simulink model "MBD_Arnav2020b"  (R2020b)
settings: Solver=FixedStepAuto  StartTime=0.0  StopTime=inf  FixedStep=1  RelTol=1e-3
undefined symbols (not defined in the file): sigbuilder_block
settings Model: Creator=99003730  LastModifiedBy=99003730

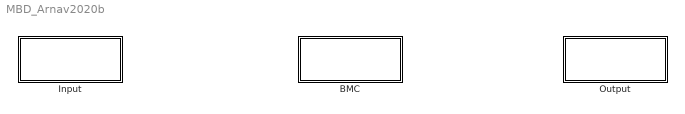
== system MBD_Arnav2020b ==
  BMC : Subsystem
  Input : Subsystem
  Output : Subsystem

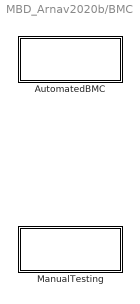
== system MBD_Arnav2020b/BMC ==
  AutomatedBMC : Subsystem
  ManualTesting : Subsystem

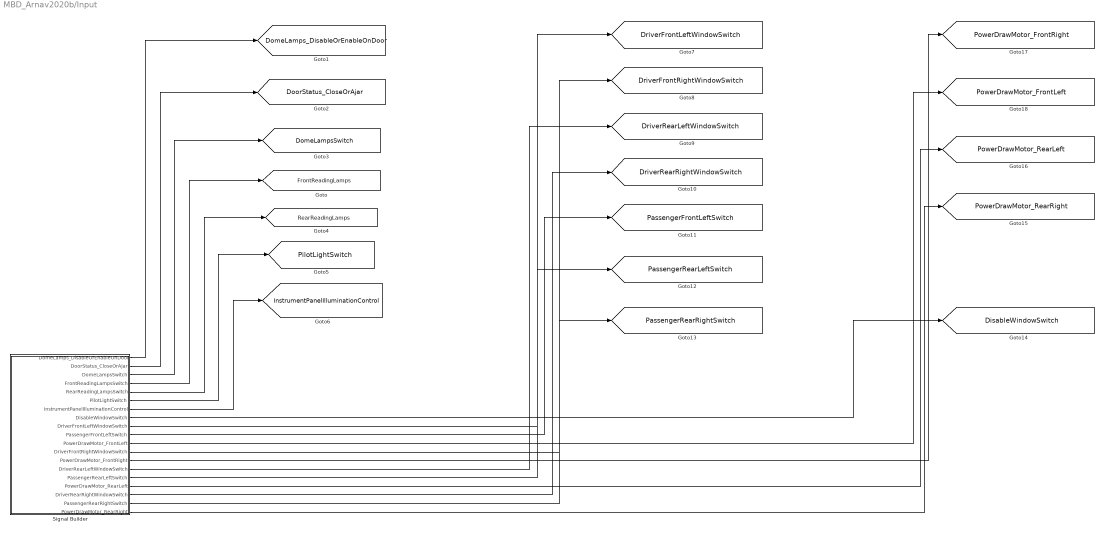
== system MBD_Arnav2020b/Input ==
  Signal Builder : Subsystem  Tag=STV Subsys  LoadFcn=sigbuilder_block('load');  StartFcn=sigbuilder_block('start');  StopFcn=sigbuilder_block('stop');  ClipboardFcn=sigbuilder_block('clipboard');  mask(Sigbuilder block){tuvar=[0:10]}
      mask help: Simulink:masks:SigbuilderBlock_MD
      mask init:
      | if ~strcmp(get_param(bdroot(gcbh),'SimulationStatus'),'stopped') tuvar = sigbuilder_block('maskInit'); end
      settings: CopyFcn=sigbuilder_block('copy');  DeleteFcn=sigbuilder_block('delete');  ModelCloseFcn=sigbuilder_block('modelClose');  PreSaveFcn=sigbuilder_block('preSave');  PauseFcn=sigbuilder_block('pause');  ContinueFcn=sigbuilder_block('continue');  NameChangeFcn=sigbuilder_block('namechange');  OpenFcn=sigbuilder_block('open',[6 80.25 1188 465.75 ]);  CloseFcn=sigbuilder_block('close');
      mask Display: plot(0, 0, 100, 100,[2, 2, 32, 32, 2], [68, 8, 8, 68, 68],[32, 2], [38, 38], [32, 19, 2],[53, 60, 44], [32, 17, 17, 2],[16, 16, 31, 31]);txt = getActiveGroup(gcbh);text(2, 100, txt,'verticalAlignment', 'top');
  tag scope: DisableWindowSwitch=global, DomeLampsSwitch=global, DomeLamps_DisableOrEnableOnDoor=global, DoorStatus_CloseOrAjar=global, DriverFrontLeftWindowSwitch=global, DriverFrontRightWindowSwitch=global, DriverRearLeftWindowSwitch=global, DriverRearRightWindowSwitch=global, FrontReadingLamps=global, InstrumentPanelIlluminationControl=global, PassengerFrontLeftSwitch=global, PassengerRearLeftSwitch=global, PassengerRearRightSwitch=global, PilotLightSwitch=global, PowerDrawMotor_FrontLeft=global, PowerDrawMotor_FrontRight=global, PowerDrawMotor_RearLeft=global, PowerDrawMotor_RearRight=global, RearReadingLamps=global
  wires:
  Signal Builder/9(DriverFrontLeftWindowSwitch) -> [DriverFrontLeftWindowSwitch]
  Signal Builder/12(DriverFrontRightWindowSwitch) -> [DriverFrontRightWindowSwitch]
  Signal Builder/14(DriverRearLeftWindowSwitch) -> [DriverRearLeftWindowSwitch]
  Signal Builder/17(DriverRearRightWindowSwitch) -> [DriverRearRightWindowSwitch]
  Signal Builder/10(PassengerFrontLeftSwitch) -> [PassengerFrontLeftSwitch]
  Signal Builder/15(PassengerRearLeftSwitch) -> [PassengerRearLeftSwitch]
  Signal Builder/18(PassengerRearRightSwitch) -> [PassengerRearRightSwitch]
  Signal Builder/13(PowerDrawMotor_FrontRight) -> [PowerDrawMotor_FrontRight]
  Signal Builder/11(PowerDrawMotor_FrontLeft) -> [PowerDrawMotor_FrontLeft]
  Signal Builder/16(PowerDrawMotor_RearLeft) -> [PowerDrawMotor_RearLeft]
  Signal Builder/19(PowerDrawMotor_RearRight) -> [PowerDrawMotor_RearRight]
  Signal Builder/8(DisableWindowSwitch) -> [DisableWindowSwitch]
  Signal Builder/1(DomeLamps_DisableOrEnableOnDoor) -> [DomeLamps_DisableOrEnableOnDoor]
  Signal Builder/2(DoorStatus_CloseOrAjar) -> [DoorStatus_CloseOrAjar]
  Signal Builder/3(DomeLampsSwitch) -> [DomeLampsSwitch]
  Signal Builder/4(FrontReadingLampsSwitch) -> [FrontReadingLamps]
  Signal Builder/5(RearReadingLampsSwitch) -> [RearReadingLamps]
  Signal Builder/6(PilotLightSwitch) -> [PilotLightSwitch]
  Signal Builder/7(InstrumentPanelIlluminationControl) -> [InstrumentPanelIlluminationControl]

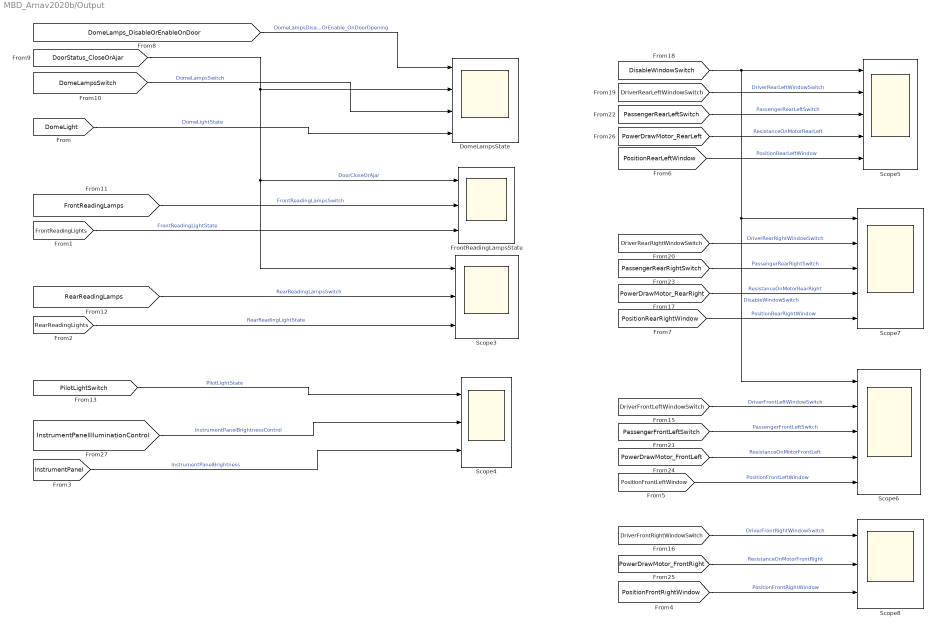
== system MBD_Arnav2020b/Output ==
  DomeLampsState : Scope  NumInputPorts=4
  FrontReadingLampsState : Scope  NumInputPorts=3
  Scope3 : Scope  NumInputPorts=3
  Scope4 : Scope  NumInputPorts=3
  Scope5 : Scope  NumInputPorts=5
  Scope6 : Scope  NumInputPorts=5
  Scope7 : Scope  NumInputPorts=5
  Scope8 : Scope  NumInputPorts=3
  wires:
  [RearReadingLights] -> Scope3/3  "RearReadingLightState"
  [FrontReadingLights] -> FrontReadingLampsState/3  "FrontReadingLightState"
  [DomeLight] -> DomeLampsState/4  "DomeLightState"
  [InstrumentPanel] -> Scope4/3  "InstrumentPanelBrightness"
  [PositionRearLeftWindow] -> Scope5/5  "PositionRearLeftWindow"
  [DomeLamps_DisableOrEnableOnDoor] -> DomeLampsState/1  "DomeLampsDisableOrEnable_OnDoorOpening"
  [DoorStatus_CloseOrAjar] -> Scope3/1, FrontReadingLampsState/1, DomeLampsState/2  "DoorCloseOrAjar"
  [DomeLampsSwitch] -> DomeLampsState/3  "DomeLampsSwitch"
  [FrontReadingLamps] -> FrontReadingLampsState/2  "FrontReadingLampsSwitch"
  [RearReadingLamps] -> Scope3/2  "RearReadingLampsSwitch"
  [PilotLightSwitch] -> Scope4/1  "PilotLightState"
  [InstrumentPanelIlluminationControl] -> Scope4/2  "InstrumentPanelBrightnessControl"
  [DisableWindowSwitch] -> Scope6/1, Scope7/1, Scope5/1  "DisableWindowSwitch"
  [DriverRearLeftWindowSwitch] -> Scope5/2  "DriverRearLeftWindowSwitch"
  [PassengerRearLeftSwitch] -> Scope5/3  "PassengerRearLeftSwitch"
  [PowerDrawMotor_RearLeft] -> Scope5/4  "ResistanceOnMotorRearLeft"
  [DriverRearRightWindowSwitch] -> Scope7/2  "DriverRearRightWindowSwitch"
  [PassengerRearRightSwitch] -> Scope7/3  "PassengerRearRightSwitch"
  [PowerDrawMotor_RearRight] -> Scope7/4  "ResistanceOnMotorRearRight"
  [PositionRearRightWindow] -> Scope7/5  "PositionRearRightWindow"
  [DriverFrontLeftWindowSwitch] -> Scope6/2  "DriverFrontLeftWindowSwitch"
  [PassengerFrontLeftSwitch] -> Scope6/3  "PassengerFrontLeftSwitch"
  [PowerDrawMotor_FrontLeft] -> Scope6/4  "ResistanceOnMotorFrontLeft"
  [PositionFrontLeftWindow] -> Scope6/5  "PositionFrontLeftWindow"
  [DriverFrontRightWindowSwitch] -> Scope8/1  "DriverFrontRightWindowSwitch"
  [PowerDrawMotor_FrontRight] -> Scope8/2  "ResistanceOnMotorFrontRight"
  [PositionFrontRightWindow] -> Scope8/3  "PositionFrontRightWindow"

== system MBD_Arnav2020b/BMC/AutomatedBMC ==
  "Arnav's Subsytem (Interior Lighting and power windows) " : Subsystem

== system MBD_Arnav2020b/BMC/ManualTesting ==
  Manual Testing Arnav : Subsystem

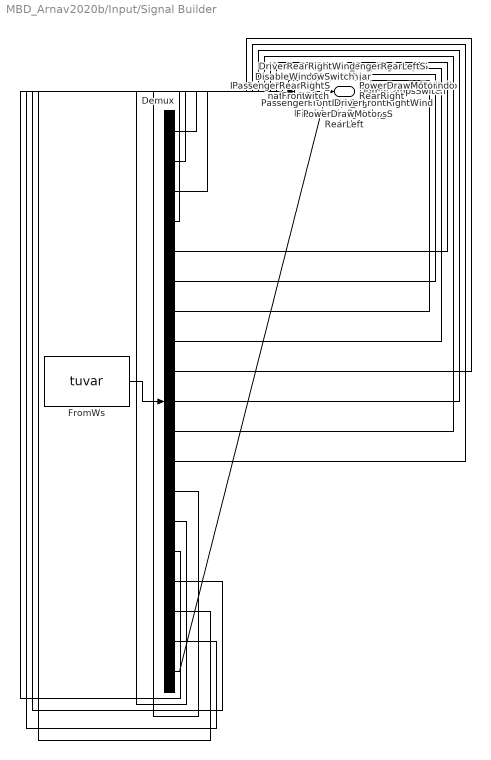
== system MBD_Arnav2020b/Input/Signal Builder ==
  Demux : Demux  Tag=STV Demux  Outputs=19
      settings: DisplayOption=none
  FromWs : FromWorkspace  Tag=STV FromWs  VariableName=tuvar  SampleTime=1
      SigBuilderData=|
      | common.afterFinalStr = 'Extrapolate'
      | common.sampleTime = '1'
      | dataSet.timeRange = [0 25]
      | dataSet.name = 'Sheet1'
      | sbobj.Name = 'Signal Builder'
      | sbobj.Groups.Name = 'Sheet1'
      | sbobj.Groups.Signals(1).Name = 'DomeLamps_DisableOrEnableOnDoor'
      | sbobj.Groups.Signals(1).XData = [0 1 2 3 4 5 6 7 8 9 10 11 12 13 14 15 16 17 18 19 20 21 22 23 24 25]
      | sbobj.Groups.Signals(1).YData = [0 0 0 0 1 1 1 1 0 0 0 0 1 1 1 1 0 0 0 0 1 1 1 1 1 0]
      | sbobj.Groups.Signals(2).Name = 'DoorStatus_CloseOrAjar'
      | sbobj.Groups.Signals(2).XData = [0 1 2 3 4 5 6 7 8 9 10 11 12 13 14 15 16 17 18 19 20 21 22 23 24 25]
      | sbobj.Groups.Signals(2).YData = [0 0 1 1 0 0 0 1 0 0 1 1 0 0 1 1 0 0 1 1 0 0 1 1 1 0]
      | sbobj.Groups.Signals(3).Name = 'DomeLampsSwitch'
      | sbobj.Groups.Signals(3).XData = [0 1 2 3 4 5 6 7 8 9 10 11 12 13 14 15 16 17 18 19 20 21 22 23 24 25]
      | sbobj.Groups.Signals(3).YData = [0 1 0 1 0 0 0 1 0 0 0 1 0 1 0 1 0 1 0 1 0 1 0 1 1 0]
      | sbobj.Groups.Signals(4).Name = 'FrontReadingLampsSwitch'
      | sbobj.Groups.Signals(4).XData = [0 1 2 3 4 5 6 7 8 9 10 11 12 13 14 15 16 17 18 19 20 21 22 23 24 25]
      | sbobj.Groups.Signals(4).YData = [0 1 0 1 0 1 0 1 0 1 0 1 0 1 0 1 0 1 0 1 0 1 0 1 0 1]
      | sbobj.Groups.Signals(5).Name = 'RearReadingLampsSwitch'
      | sbobj.Groups.Signals(5).XData = [0 1 2 3 4 5 6 7 8 9 10 11 12 13 14 15 16 17 18 19 20 21 22 23 24 25]
      | sbobj.Groups.Signals(5).YData = [0 1 0 1 0 1 0 1 0 1 0 1 0 1 0 1 0 1 0 1 0 1 0 1 0 1]
      | sbobj.Groups.Signals(6).Name = 'PilotLightSwitch'
      | sbobj.Groups.Signals(6).XData = [0 1 2 3 4 5 6 7 8 9 10 11 12 13 14 15 16 17 18 19 20 21 22 23 24 25]
      | sbobj.Groups.Signals(6).YData = [0 0 0 0 0 0 0 0 0 0 1 1 1 1 1 1 1 1 1 1 0 0 0 0 0 0]
      | sbobj.Groups.Signals(7).Name = 'InstrumentPanelIlluminationControl'
      | sbobj.Groups.Signals(7).XData = [0 1 2 3 4 5 6 7 8 9 10 11 12 13 14 15 16 17 18 19 20 21 22 23 24 25]
      | sbobj.Groups.Signals(7).YData = [1 2 3 4 5 6 7 8 9 10 1 2 3 4 5 6 7 8 9 10 1 2 3 4 5 6]
      | sbobj.Groups.Signals(8).Name = 'DisableWindowSwitch'
      | sbobj.Groups.Signals(8).XData = [0 1 2 3 4 5 6 7 8 9 10 11 12 13 14 15 16 17 18 19 20 21 22 23 24 25]
      | sbobj.Groups.Signals(8).YData = [0 0 0 0 0 0 0 0 0 0 0 0 0 0 0 0 0 1 1 0 1 1 1 0 0 0]
      | sbobj.Groups.Signals(9).Name = 'DriverFrontLeftWindowSwitch'
      | sbobj.Groups.Signals(9).XData = [0 1 2 3 4 5 6 7 8 9 10 11 12 13 14 15 16 17 18 19 20 21 22 23 24 25]
      | sbobj.Groups.Signals(9).YData = [1 1 1 0 0 0 0 0 -1 -1 -1 0 0 2 0 0 0 0 -2 0 0 0 0 0 1 0]
      | sbobj.Groups.Signals(10).Name = 'PassengerFrontLeftSwitch'
      | sbobj.Groups.Signals(10).XData = [0 1 2 3 4 5 6 7 8 9 10 11 12 13 14 15 16 17 18 19 20 21 22 23 24 25]
      | sbobj.Groups.Signals(10).YData = [0 -1 -1 1 1 1 -1 -1 0 0 0 0 0 0 0 -2 1 2 0 2 1 1 0 2 0 0]
      | sbobj.Groups.Signals(11).Name = 'PowerDrawMotor_FrontLeft'
      | sbobj.Groups.Signals(11).XData = [0 1 2 3 4 5 6 7 8 9 10 11 12 13 14 15 16 17 18 19 20 21 22 23 24 25]
      | sbobj.Groups.Signals(11).YData = [2 2 2 2 2 2 2 2 2 2 2 2 2 2 2 2 2 2 2 2 2 4 1 1 1 1]
      | sbobj.Groups.Signals(12).Name = 'DriverFrontRightWindowSwitch'
      | sbobj.Groups.Signals(12).XData = [0 1 2 3 4 5 6 7 8 9 10 11 12 13 14 15 16 17 18 19 20 21 22 23 24 25]
      | sbobj.Groups.Signals(12).YData = [1 1 1 1 1 0 0 0 -1 -1 -1 0 0 2 0 0 0 0 -2 0 0 0 0 1 2 0]
      | sbobj.Groups.Signals(13).Name = 'PowerDrawMotor_FrontRight'
      | sbobj.Groups.Signals(13).XData = [0 1 2 3 4 5 6 7 8 9 10 11 12 13 14 15 16 17 18 19 20 21 22 23 24 25]
      | sbobj.Groups.Signals(13).YData = [2 2 2 2 2 2 2 2 2 2 2 2 2 2 2 2 2 2 2 2 2 4 1 1 1 1]
      | sbobj.Groups.Signals(14).Name = 'DriverRearLeftWindowSwitch'
      | sbobj.Groups.Signals(14).XData = [0 1 2 3 4 5 6 7 8 9 10 11 12 13 14 15 16 17 18 19 20 21 22 23 24 25]
      | sbobj.Groups.Signals(14).YData = [1 1 1 0 0 0 0 0 -1 -1 -1 0 0 2 0 0 0 0 -2 0 0 0 0 0 0 0]
      | sbobj.Groups.Signals(15).Name = 'PassengerRearLeftSwitch'
      | sbobj.Groups.Signals(15).XData = [0 1 2 3 4 5 6 7 8 9 10 11 12 13 14 15 16 17 18 19 20 21 22 23 24 25]
      | sbobj.Groups.Signals(15).YData = [0 -1 -1 1 1 1 -1 -1 0 0 0 0 0 0 0 -2 1 2 0 2 1 1 0 2 0 0]
      | sbobj.Groups.Signals(16).Name = 'PowerDrawMotor_RearLeft'
      | sbobj.Groups.Signals(16).XData = [0 1 2 3 4 5 6 7 8 9 10 11 12 13 14 15 16 17 18 19 20 21 22 23 24 25]
      | sbobj.Groups.Signals(16).YData = [2 2 2 2 2 2 2 2 2 2 2 2 2 2 2 2 2 2 2 2 2 4 1 1 1 1]
      | sbobj.Groups.Signals(17).Name = 'DriverRearRightWindowSwitch'
      | sbobj.Groups.Signals(17).XData = [0 1 2 3 4 5 6 7 8 9 10 11 12 13 14 15 16 17 18 19 20 21 22 23 24 25]
      | sbobj.Groups.Signals(17).YData = [1 1 1 0 0 0 0 0 -1 -1 -1 0 0 2 0 0 0 0 -2 0 0 0 0 0 0 0]
      | sbobj.Groups.Signals(18).Name = 'PassengerRearRightSwitch'
      | sbobj.Groups.Signals(18).XData = [0 1 2 3 4 5 6 7 8 9 10 11 12 13 14 15 16 17 18 19 20 21 22 23 24 25]
      | sbobj.Groups.Signals(18).YData = [0 -1 -1 1 1 1 -1 -1 0 0 0 0 0 0 0 -2 1 2 0 2 1 1 0 2 0 0]
      | sbobj.Groups.Signals(19).Name = 'PowerDrawMotor_RearRight'
      | sbobj.Groups.Signals(19).XData = [0 1 2 3 4 5 6 7 8 9 10 11 12 13 14 15 16 17 18 19 20 21 22 23 24 25]
      | sbobj.Groups.Signals(19).YData = [2 2 2 4 2 2 2 2 2 2 2 2 2 2 2 2 2 2 4 2 2 4 1 1 1 1]
      | sbobj.Groups.TimeRange = [0 25]
  DomeLamps_DisableOrEnableOnDoor : Outport  Tag=STV Outport
  DoorStatus_CloseOrAjar : Outport  Tag=STV Outport  Port=2
  DomeLampsSwitch : Outport  Tag=STV Outport  Port=3
  FrontReadingLampsSwitch : Outport  Tag=STV Outport  Port=4
  RearReadingLampsSwitch : Outport  Tag=STV Outport  Port=5
  PilotLightSwitch : Outport  Tag=STV Outport  Port=6
  InstrumentPanelIlluminationControl : Outport  Tag=STV Outport  Port=7
  DisableWindowSwitch : Outport  Tag=STV Outport  Port=8
  DriverFrontLeftWindowSwitch : Outport  Tag=STV Outport  Port=9
  PassengerFrontLeftSwitch : Outport  Tag=STV Outport  Port=10
  PowerDrawMotor_FrontLeft : Outport  Tag=STV Outport  Port=11
  DriverFrontRightWindowSwitch : Outport  Tag=STV Outport  Port=12
  PowerDrawMotor_FrontRight : Outport  Tag=STV Outport  Port=13
  DriverRearLeftWindowSwitch : Outport  Tag=STV Outport  Port=14
  PassengerRearLeftSwitch : Outport  Tag=STV Outport  Port=15
  PowerDrawMotor_RearLeft : Outport  Tag=STV Outport  Port=16
  DriverRearRightWindowSwitch : Outport  Tag=STV Outport  Port=17
  PassengerRearRightSwitch : Outport  Tag=STV Outport  Port=18
  PowerDrawMotor_RearRight : Outport  Tag=STV Outport  Port=19
  wires:
  FromWs/1 -> Demux/1
  Demux/1 -> DomeLamps_DisableOrEnableOnDoor/1
  Demux/2 -> DoorStatus_CloseOrAjar/1
  Demux/3 -> DomeLampsSwitch/1
  Demux/4 -> FrontReadingLampsSwitch/1
  Demux/5 -> RearReadingLampsSwitch/1
  Demux/6 -> PilotLightSwitch/1
  Demux/7 -> InstrumentPanelIlluminationControl/1
  Demux/8 -> DisableWindowSwitch/1
  Demux/9 -> DriverFrontLeftWindowSwitch/1
  Demux/10 -> PassengerFrontLeftSwitch/1
  Demux/11 -> PowerDrawMotor_FrontLeft/1
  Demux/12 -> DriverFrontRightWindowSwitch/1
  Demux/13 -> PowerDrawMotor_FrontRight/1
  Demux/14 -> DriverRearLeftWindowSwitch/1
  Demux/15 -> PassengerRearLeftSwitch/1
  Demux/16 -> PowerDrawMotor_RearLeft/1
  Demux/17 -> DriverRearRightWindowSwitch/1
  Demux/18 -> PassengerRearRightSwitch/1
  Demux/19 -> PowerDrawMotor_RearRight/1

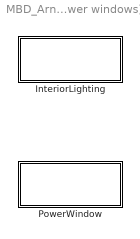
== system MBD_Arnav2020b/BMC/AutomatedBMC/Arnav's Subsytem (Interior Lighting and power windows)  ==
  " InteriorLighting" : Subsystem
  PowerWindow : Subsystem

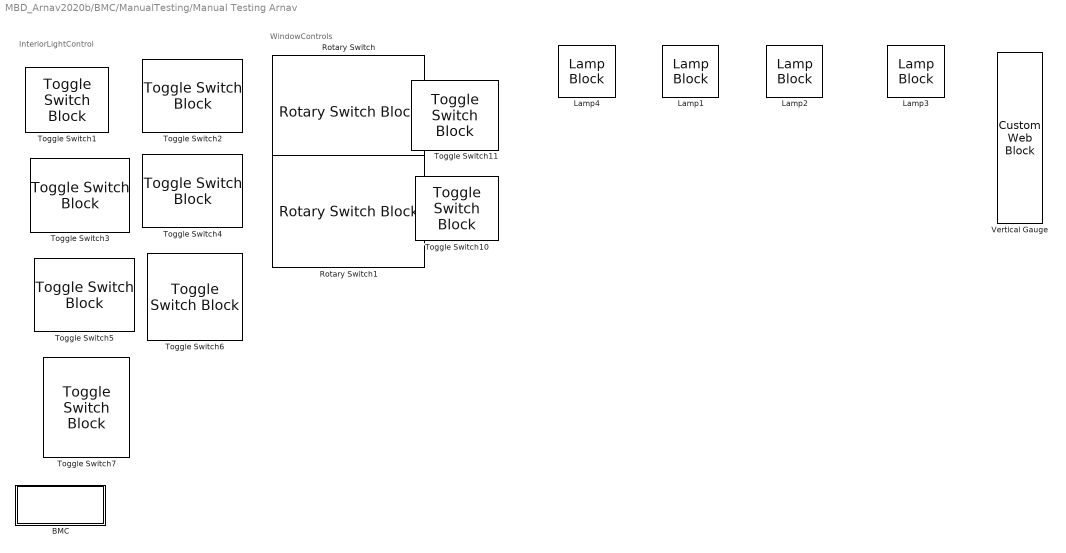
== system MBD_Arnav2020b/BMC/ManualTesting/Manual Testing Arnav ==
  note: WindowControls
  note: InteriorLightControl
  BMC : Subsystem
  Lamp{1..4} (4 alike) : LampBlock
  Rotary Switch : RotarySwitchBlock
      settings: Values={{'Off', 'Down', 'Express Down', 'Up', 'Express Up'}, [0 -1 -2 1 2]}
  Rotary Switch1 : RotarySwitchBlock
      settings: Values={{'Off', 'Down', 'Express Down', 'Up', 'Express Up'}, [0 -1 -2 1 2]}
  Toggle Switch{1..7,10..11} (9 alike) : ToggleSwitchBlock
  Vertical Gauge : CustomWebBlock  ShowInitialText=on  Configuration="{\"components\":[{\"name\":\"LinearScaleComponent\",\"settings\":{\"bounds\":{\"max\":5,\"min\":0,\"tickInterval\":\"auto\"},\"internalTickHeightScaleFactor\":0.5,\"labelColor\":[250,245,199],\"labelFont\":{\"font\":\"Arial\",\"fontSize\":12},\"labelTransparency\":1,\"needleImage\":{\"size\":[21,75],\"src\":\"data:image\\/svg+xml;base64,PHN2ZyB4bWxucz0iaHR0cDovL3d3dy53My5vcmcvMjAwMC9zdmciIHhtbG5zOnhsaW5rPSJodHRwOi8vd3d3LnczLm9yZy8xOTk5L3hsaW5rIiB2aWV3Qm94PSIwIDAgMjEgNzUiPjxkZWZzPjxzdHlsZT4uY2xzLTF7ZmlsbDpub25lO30uY2xzLTJ7aXNvbGF0aW9uOmlzb2xhdGU7fS5jbHMtM3tjbGlwLXBhdGg6dXJsKCNjbGlwLXBhdGgpO30uY2xzLTR7b3BhY2l0eTowLjM7bWl4LWJsZW5kLW1vZGU6bXVsdGlwbHk7fS5jbHMtNXtmaWxsOiNlYjI2Mjk7fTwvc3R5bGU+PGNsaXBQYXRoIGlkPSJjbGlwLXBhdGgiIHRyYW5zZm9y ...(+1928 chars)\",\"srcOrientation\":\"horizontal\"},\"needleOffset\":[-0.01094391244870041,0],\"needleSize\":{\"height\":0.11960078534031414,\"width\":0.7589285714285714},\"position\":[0.015887605042016806,0.06986607142857143,0.8,0.9641544117647058],\"scaleColors\":[],\"scaleColorsSize\":0.2,\"showLabels\":1,\"showMinorTicks\":0,\"showSpanLine\":1,\"showTicks\":1,\"tickColor\":[250,245,200],\"tickTransparency\":1,\"valueBarColor\":[23,89,176],\"valueBarOffset\":0,\"valueBarSize\":0.23,\"valueBarTransparency\":1}},{\"name\":\"BackgroundImageComponent\",\"settings\":{\"image\":{\"size\":[101,380],\"src\":\"data:image\\/svg+xml;base64,PHN2ZyB4bWxucz0iaHR0cDovL3d3dy53My5vcmcvMjAwMC9zdmciIHZpZXdCb3g9IjAgMCAxMDEgMzgwIj48ZGVmcz48c3R5bGU+LmNscy0xe2ZpbGw6IzAwMmI0Mjt9LmNscy0ye2ZpbGw6IzQyNzA4Mjt9LmNscy0ze2ZpbGw6IzdjYTBiMjt9PC9zdHlsZT48L2RlZnM+PHRpdGxlPnZlcnRpY2FsX2dhdWdlX2JhY2tncm91bmRfMTwvdGl0bGU+PGcgaWQ9IkxheWVyXzIiIGRhdGEtbmFtZT0iTGF5ZXIgMiI+PGcgaWQ9IkxheWVyXzEtMiIgZGF0YS1uYW1lPSJMYXllciAxIj48cmVjdCBjbGFzcz0iY2xzLTEiIHg9IjExIiB5PSIxMSIgd2lkdGg9Ijc5IiBoZWlnaHQ9IjM1OCIvPjxwYXRoIGNsYXNzPSJjbHMtMiIgZD0iTTkzLDhIOFYzNzJIOTNaTTExLDM2OVYxMUg5MFYzNjlaIi8+PHBhdGggY2xhc3M9ImNscy0zIiBkPSJNMTAxLDBIMFYzODBIMTAxWk04LDM3MlY4SDkzVjM3MloiLz48L2c+PC9nPjwvc3ZnPg==\",\"srcOrientation\":\"vertical\"},\"position\":[0,0,1,1],\"scaleMode\":\"0\"}},{\"name\":\"ForegroundImageComponent\",\"settings\":{\"image\":{\"size\":[0,0],\"src\":\"default\",\"srcOrientation\":[]},\"isForeground\":1,\"position\":[0,0,1,1],\"scaleMode\":\"0\"}}],\"settings\":{\"BindingType\":\"signal\",\"aspectRatio\":0.2647058823529412,\"fixedAspectRatio\":\"on\",\"orientation\":\"vertical\"},\"type\":\"LinearGauge\"}"

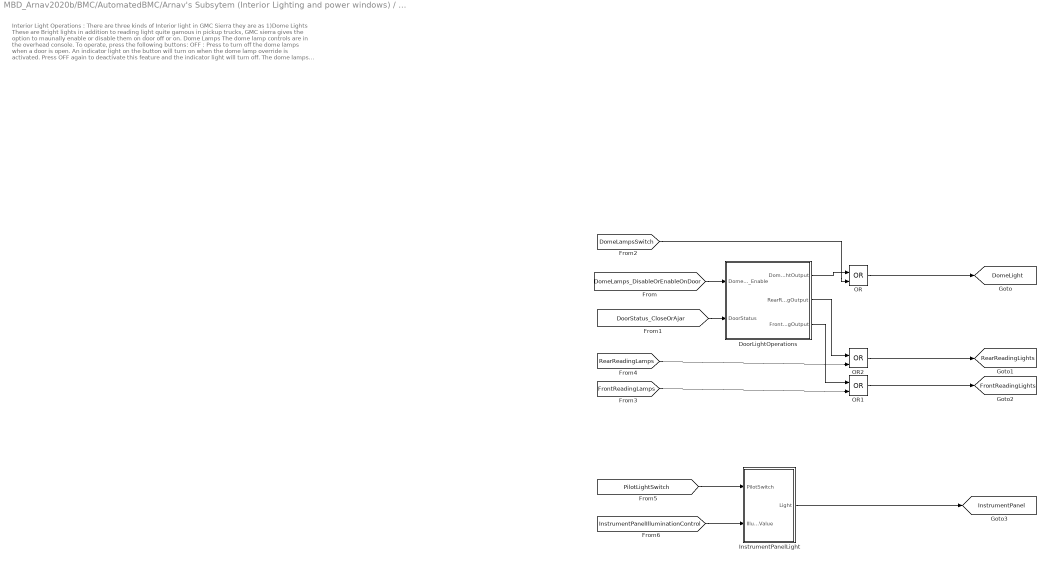
== system MBD_Arnav2020b/BMC/AutomatedBMC/Arnav's Subsytem (Interior Lighting and power windows) / InteriorLighting ==
  note: Interior Light Operations :
      | There are three kinds of Interior light in GMC Sierra they are as
      | 1)Dome Lights
      |
      | These are Bright lights in addition to reading light quite gamous in pickup trucks, GMC sierra gives the option to maunally enable or disable them on door off or on.
      |
      | Dome Lamps The dome lamp controls are in the overhead console. To operate, press the following buttons: OFF : Press to turn off the dome lamps when a door is open. An indicator light on the button will turn on when the dome lamp override is activated. Press OFF again to deactivate this feature and the indicator light will turn off. The dome lamps will come on when doors are opened.
      |
      | Source: GMC Sierra/Sierra Denali Owner Manual (GMNA-Localizing-U.S./Canada/ Mexico-13337776) - 2020 - CRC - 8/27/19
      |
      | 2)Reading Lamps
      |
      | The regular reading lamps present in everycar which are enabled on pressing.
      | Reading Lamps There are reading lamps on the overhead console and over the rear seats. These lamps come on when any door is opened. Front Reading Lamps The front reading lamps are in the overhead console. Press the lamp lenses to turn the front reading lamps on or off. Rear Reading Lamps The rear reading lamps are over the rear seats. Press the lamp lens to turn the rear reading lamps on or off.
      | Source:: GMC Sierra/Sierra Denali Owner Manual (GMNA-Localizing-U.S./Canada/ Mexico-13337776) - 2020 - CRC - 8/27/19
      | 3)Instrument Panel:
      |
      | GMC Sierra Gives an option to control the brightness of instrument panel which is implemented here, it is turned on only when pilot lights are turned on
      |
      | Instrument Panel Illumination Control This feature controls the brightness of the steering wheel and instrument panel lights. The instrument panel illumination control is next to the exterior lamp control. D : Press D + to brighten or D − to dim the lights.
      | Source:: GMC Sierra/Sierra Denali Owner Manual (GMNA-Localizing-U.S./Canada/ Mexico-13337776) - 2020 - CRC - 8/27/19
  DoorLightOperations : Stateflow chart  TreatAsAtomicUnit=on
      settings: PortSchema="{\"entries\":[{\"content\":{\"sides\":[{\"content\":{\"connectorIds\":[\"In1\",\"In2\"]},\"type\":\"ConnectorPlacement.EquallySpacedRectSide\",\"uuid\":\"88cb4188-67b2-46bf-b15b-06b49d8edfa4\"},{\"content\":{\"connectorIds\":[\"Out3\",\"Out2\",\"Out1\"],\"side\":\"RIGHT\"},\"type\":\"ConnectorPlacement.EquallySpacedRectSide\",\"uuid\":\"9065dfda-8219-4130-8b57-23394e2d071b\"},{\"content\":{\"connectorIds\":[],\"side\":\"TOP\"},\"type\":\"ConnectorPlacement.EquallySpacedRectSide\",\"uuid\":\"33c36138-f19b-46a2-8d7c-63d89e2c1b86\"},{\"content\":{\"connectorIds\":[],\"side\":\"BOTTOM\"},\"type\":\"ConnectorPlacement.EquallySpacedRectSide\",\"uuid\":\"55cb48c3-7f99-4974-9ce7-6609371a2e27\"},{\"content\":{\"connectorIds\":[],\"side\":\"HIDDEN\"},\"type\":\"ConnectorPlacement.EquallySpacedRectSide\",\"uuid\":\"670a4799-206d-49f1-9ba7-7022d4fdbb0d\"}]},\"type\":\"ConnectorPlacement.EquallySpacedConnector\",\"uuid\":\"df8b59d8-5929-4621-bd40-717753a9fdb2\"}],\"packageUris\":[\"http://schema.mathworks.com/mf0/Connector/R2020b\"],\"version\":\"1.0\"}"
  InstrumentPanelLight : Stateflow chart  TreatAsAtomicUnit=on
  OR : Logic  Operator=OR  IconShape=distinctive  AllPortsSameDT=off  OutDataTypeStr=boolean
  OR1 : Logic  Operator=OR  IconShape=distinctive  AllPortsSameDT=off  OutDataTypeStr=boolean
  OR2 : Logic  Operator=OR  IconShape=distinctive  AllPortsSameDT=off  OutDataTypeStr=boolean
  tag scope: DomeLight=global, FrontReadingLights=global, InstrumentPanel=global, RearReadingLights=global
  wires:
  OR1/1 -> [FrontReadingLights]
  OR2/1 -> [RearReadingLights]
  OR/1 -> [DomeLight]
  DoorLightOperations/3(DomeLightOutput) -> OR/1
  DoorLightOperations/2(RearReadingOutput) -> OR2/1
  DoorLightOperations/1(FrontReadingOutput) -> OR1/1
  [FrontReadingLamps] -> OR1/2
  [DomeLampsSwitch] -> OR/2
  [RearReadingLamps] -> OR2/2
  [DoorStatus_CloseOrAjar] -> DoorLightOperations/2(DoorStatus)
  [DomeLamps_DisableOrEnableOnDoor] -> DoorLightOperations/1(DomeLight_Enable)
  [PilotLightSwitch] -> InstrumentPanelLight/1(PilotSwitch)
  [InstrumentPanelIlluminationControl] -> InstrumentPanelLight/2(IlluminationValue)
  InstrumentPanelLight/1(Light) -> [InstrumentPanel]

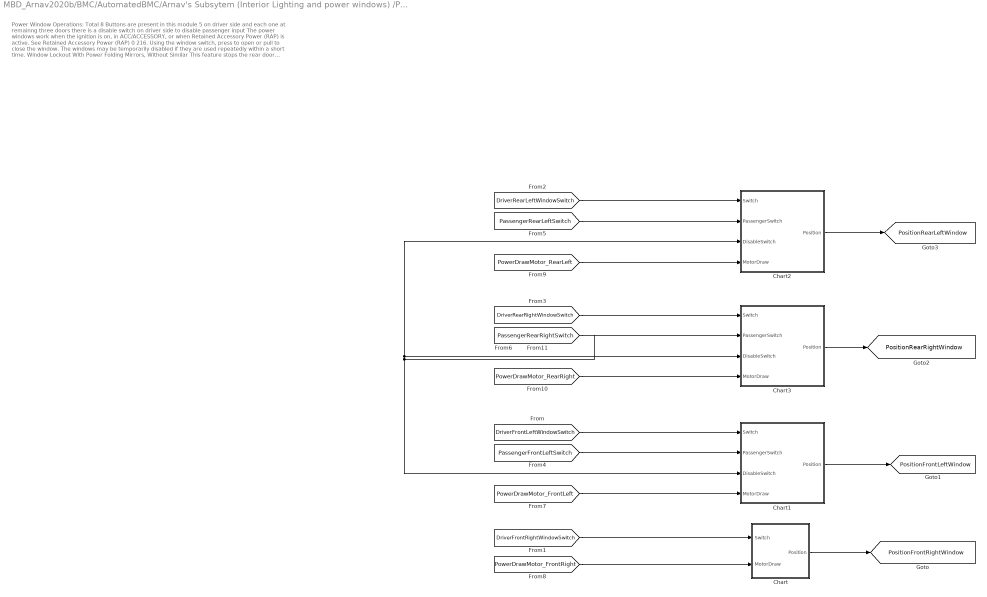
== system MBD_Arnav2020b/BMC/AutomatedBMC/Arnav's Subsytem (Interior Lighting and power windows) /PowerWindow ==
  note: Power Window Operations:
      |
      | Total 8 Buttons are present in this module
      | 5 on driver side and each one at remainng three doors
      | there is a disable switch on driver side to disable passenger input
      |
      | The power windows work when the ignition is on, in ACC/ACCESSORY, or when Retained Accessory Power (RAP) is active. See Retained Accessory Power (RAP) 0 216. Using the window switch, press to open or pull to close the window. The windows may be temporarily disabled if they are used repeatedly within a short time. Window Lockout With Power Folding Mirrors, Without Similar This feature stops the rear door passenger window switches from working except from the driver position. Press 2 to engage the rear window lockout feature. The indicator light is on when engaged. Press 2 again to disengage. Windows Express Movement All windows can be opened without holding the window switch. Press the switch down fully and quickly release to express open the window. If equipped, pull the window switch up fully and quickly release to express close the window. Briefly press or pull the window switch in the same direction to stop that window’s express movement. Express Window Down L: If equipped, this button will be on the center stack. Press and hold L to open all windows. Release L to stop all movement. Use the power window switches to close each window. Window Automatic Reversal System The express-close feature will reverse window movement if it comes in contact with an object.GMC Sierra/Sierra Denali Owner Manual (GMNA-Localizing-U.S./Canada/ Mexico-13337776) - 2020 - CRC - 8/27/19 Keys, Doors, and Windows 49 Extreme cold or ice could cause the window to auto-reverse. The window will operate normally after the object or condition is removed. Automatic Reversal System Override { Warning If automatic reversal system override is active, the window will not reverse automatically. You or others could be injured and the window could be damaged. Before using automatic reversal system override, make sure that all people and obstructions are clear of the window path. When the engine is on, override the automatic reversal system by pulling and holding the window switch if conditions prevent it from closing. Programming the Power Windows Programming may be necessary if the vehicle battery has been disconnected or discharged. If the window is unable to express-up, program each express-close window: 1. Close all doors. 2. Turn the ignition on or to ACC/ ACCESSORY. 3. Partially open the window to be programmed. Then close it and continue to pull the switch briefly after the window has fully closed. 4. Open the window and continue to press the switch briefly after the window has fully opened. Remote Window Operation If equipped, this feature allows the windows to be opened remotely. If enabled in vehicle personalization, press and hold K on the RKE transmitter. See Vehicle Personalization 0 156. Rear Windows Power Sliding Rear Window If equipped, the power sliding rear window works when the ignition has been turned on or to ACC/ ACCESSORY, or Retained Accessory Power (RAP) must be active. See Retained Accessory Power (RAP) 0 216. . Press the switch to open the window. . Pull the switch to close the window.
  Chart : Stateflow chart  TreatAsAtomicUnit=on
  Chart1 : Stateflow chart  TreatAsAtomicUnit=on
  Chart2 : Stateflow chart  TreatAsAtomicUnit=on
  Chart3 : Stateflow chart  TreatAsAtomicUnit=on
  tag scope: PositionFrontLeftWindow=global, PositionFrontRightWindow=global, PositionRearLeftWindow=global, PositionRearRightWindow=global
  wires:
  [DisableWindowSwitch] -> Chart3/3(DisableSwitch), Chart2/3(DisableSwitch), Chart1/3(DisableSwitch)
  [PowerDrawMotor_RearRight] -> Chart3/4(MotorDraw)
  [PassengerFrontLeftSwitch] -> Chart1/2(PassengerSwitch)
  Chart/1(Position) -> [PositionFrontRightWindow]
  [PassengerRearRightSwitch] -> Chart3/2(PassengerSwitch)
  [PowerDrawMotor_RearLeft] -> Chart2/4(MotorDraw)
  [DriverRearLeftWindowSwitch] -> Chart2/1(Switch)
  [PassengerRearLeftSwitch] -> Chart2/2(PassengerSwitch)
  [DriverFrontLeftWindowSwitch] -> Chart1/1(Switch)
  [PowerDrawMotor_FrontLeft] -> Chart1/4(MotorDraw)
  [DriverRearRightWindowSwitch] -> Chart3/1(Switch)
  Chart1/1(Position) -> [PositionFrontLeftWindow]
  [DriverFrontRightWindowSwitch] -> Chart/1(Switch)
  [PowerDrawMotor_FrontRight] -> Chart/2(MotorDraw)
  Chart2/1(Position) -> [PositionRearLeftWindow]
  Chart3/1(Position) -> [PositionRearRightWindow]

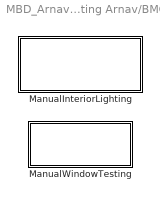
== system MBD_Arnav2020b/BMC/ManualTesting/Manual Testing Arnav/BMC ==
  ManualInteriorLighting : Subsystem
  ManualWindowTesting : Subsystem

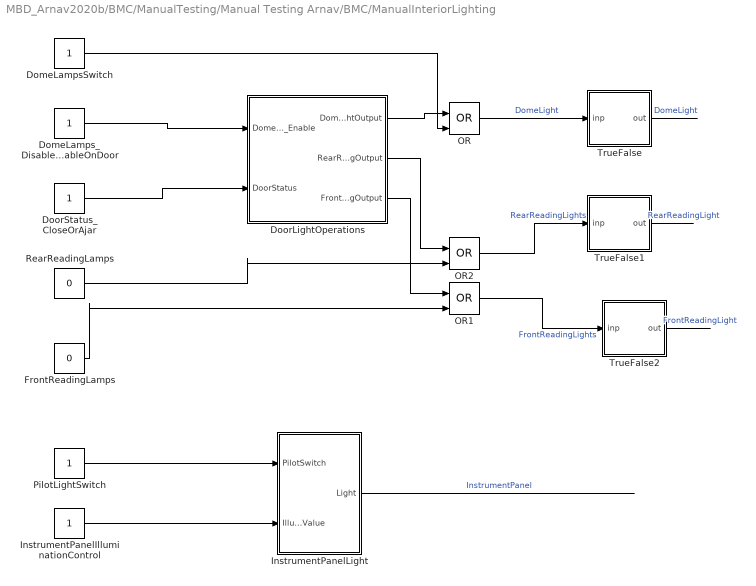
== system MBD_Arnav2020b/BMC/ManualTesting/Manual Testing Arnav/BMC/ManualInteriorLighting ==
  DomeLampsSwitch : Constant
  DomeLamps_DisableOrEnableOnDoor : Constant
  DoorLightOperations : Stateflow chart  TreatAsAtomicUnit=on
      settings: PortSchema="{\"entries\":[{\"content\":{\"sides\":[{\"content\":{\"connectorIds\":[\"In1\",\"In2\"]},\"type\":\"ConnectorPlacement.EquallySpacedRectSide\",\"uuid\":\"88cb4188-67b2-46bf-b15b-06b49d8edfa4\"},{\"content\":{\"connectorIds\":[\"Out3\",\"Out2\",\"Out1\"],\"side\":\"RIGHT\"},\"type\":\"ConnectorPlacement.EquallySpacedRectSide\",\"uuid\":\"9065dfda-8219-4130-8b57-23394e2d071b\"},{\"content\":{\"connectorIds\":[],\"side\":\"TOP\"},\"type\":\"ConnectorPlacement.EquallySpacedRectSide\",\"uuid\":\"33c36138-f19b-46a2-8d7c-63d89e2c1b86\"},{\"content\":{\"connectorIds\":[],\"side\":\"BOTTOM\"},\"type\":\"ConnectorPlacement.EquallySpacedRectSide\",\"uuid\":\"55cb48c3-7f99-4974-9ce7-6609371a2e27\"},{\"content\":{\"connectorIds\":[],\"side\":\"HIDDEN\"},\"type\":\"ConnectorPlacement.EquallySpacedRectSide\",\"uuid\":\"670a4799-206d-49f1-9ba7-7022d4fdbb0d\"}]},\"type\":\"ConnectorPlacement.EquallySpacedConnector\",\"uuid\":\"df8b59d8-5929-4621-bd40-717753a9fdb2\"}],\"packageUris\":[\"http://schema.mathworks.com/mf0/Connector/R2020b\"],\"version\":\"1.0\"}"
  DoorStatus_CloseOrAjar : Constant
  FrontReadingLamps : Constant  Value=0
  InstrumentPanelIlluminationControl : Constant
  InstrumentPanelLight : Stateflow chart  TreatAsAtomicUnit=on
  OR : Logic  Operator=OR  IconShape=distinctive  AllPortsSameDT=off  OutDataTypeStr=boolean
  OR1 : Logic  Operator=OR  IconShape=distinctive  AllPortsSameDT=off  OutDataTypeStr=boolean
  OR2 : Logic  Operator=OR  IconShape=distinctive  AllPortsSameDT=off  OutDataTypeStr=boolean
  PilotLightSwitch : Constant
  RearReadingLamps : Constant  Value=0
  TrueFalse : Stateflow chart  TreatAsAtomicUnit=on
  TrueFalse1 : Stateflow chart  TreatAsAtomicUnit=on
  TrueFalse2 : Stateflow chart  TreatAsAtomicUnit=on
  wires:
  DoorLightOperations/3(DomeLightOutput) -> OR/1
  DoorLightOperations/2(RearReadingOutput) -> OR2/1
  TrueFalse1/1(out) -> ?  "RearReadingLight"
  OR/1 -> TrueFalse/1(inp)  "DomeLight"
  TrueFalse/1(out) -> ?  "DomeLight"
  OR2/1 -> TrueFalse1/1(inp)  "RearReadingLights"
  TrueFalse2/1(out) -> ?  "FrontReadingLight"
  PilotLightSwitch/1 -> InstrumentPanelLight/1(PilotSwitch)
  DoorStatus_CloseOrAjar/1 -> DoorLightOperations/2(DoorStatus)
  DomeLamps_DisableOrEnableOnDoor/1 -> DoorLightOperations/1(DomeLight_Enable)
  OR1/1 -> TrueFalse2/1(inp)  "FrontReadingLights"
  DomeLampsSwitch/1 -> OR/2
  FrontReadingLamps/1 -> OR1/2
  RearReadingLamps/1 -> OR2/2
  InstrumentPanelIlluminationControl/1 -> InstrumentPanelLight/2(IlluminationValue)
  InstrumentPanelLight/1(Light) -> ?  "InstrumentPanel"
  DoorLightOperations/1(FrontReadingOutput) -> OR1/1

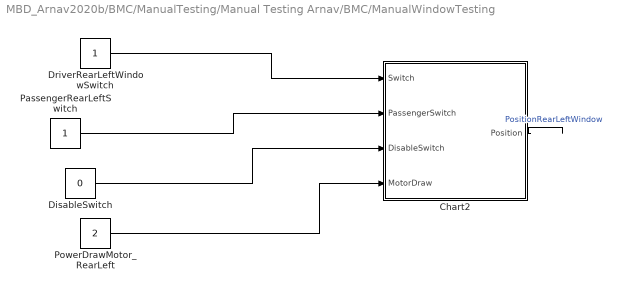
== system MBD_Arnav2020b/BMC/ManualTesting/Manual Testing Arnav/BMC/ManualWindowTesting ==
  Chart2 : Stateflow chart  TreatAsAtomicUnit=on
  DisableSwitch : Constant  Value=0
  DriverRearLeftWindowSwitch : Constant
  PassengerRearLeftSwitch : Constant
  PowerDrawMotor_RearLeft : Constant  Value=2
  wires:
  PowerDrawMotor_RearLeft/1 -> Chart2/4(MotorDraw)
  DisableSwitch/1 -> Chart2/3(DisableSwitch)
  Chart2/1(Position) -> ?  "PositionRearLeftWindow"
  DriverRearLeftWindowSwitch/1 -> Chart2/1(Switch)
  PassengerRearLeftSwitch/1 -> Chart2/2(PassengerSwitch)

== stateflow chart MBD_Arnav2020b/BMC/ManualTesting/Manual Testing Arnav/BMC/ManualInteriorLighting/TrueFalse2 ==
  state TrueFalse
    during:
    if inp==true
    out=1;
    elseif inp == false
    out=0;
    end
  (default) -> TrueFalse
  data: out output; inp input

== stateflow chart MBD_Arnav2020b/BMC/ManualTesting/Manual Testing Arnav/BMC/ManualWindowTesting/Chart2 ==
  state ExpressUp
    during:
    if Position<MaxPos && (Switch ~= -1 || Switch ~=-2 || PassengerSwitch ~=-1 || PassengerSwitch~=-2)
    Position=Position+1;
    else
    ReturnToInitial=1;
    end
    exit:
    ReturnToInitial=0;
  state WindowDown
    during:
    if Position>MinPos
    Position=Position-1;
    else
    Switche=0;
    end
    exit:
    Switche=-1;
  state Start
  state WindowUp
    during:
    if Position<MaxPos
    Position=Position+1;
    else
    Switche=0;
    end
    exit:
    Switche=1;
  state EmergencyStop
    during:
    if Position>MinPos
    Position=Position-1;
    else
    ReturnToInitial =-1;
    end
  state ExpressDown
    during:
    if Position>MinPos && (Switch~= 1 || Switch ~=2 || PassengerSwitch ~=1 || PassengerSwitch~=2)
    Position=Position-1;
    else
    ReturnToInitial =-1;
    end
    exit:
    ReturnToInitial=0;
  ExpressUp -> EmergencyStop [order 1] : [MotorDraw>3]
  Start -> ExpressUp [order 7] : [PassengerSwitch==2 && Position<MaxPos && DisableSwitch==0]
  ExpressUp -> Start [order 2] : [ReturnToInitial==1]
  Start -> ExpressUp [order 3] : [Switch==2&& Position<=MaxPos]
  Start -> EmergencyStop [order 9] : [MotorDraw>3]
  (default) -> Start
  Start -> WindowUp [order 5] : [PassengerSwitch==1 && Position<MaxPos && DisableSwitch==0]
  WindowDown -> Start [order 2] : [Switche==0]
  Start -> WindowUp [order 1] : [Switch == 1&& Position<=MaxPos]
  WindowUp -> Start [order 2] : [(Switch == 0||Switch == -1 || Switch ==-2)&&(PassengerSwitch==0||PassengerSwitch==-1||PassengerSwitch==-2)]
  Start -> WindowDown [order 2] : [Switch==-1&& Position>=MinPos ]
  WindowDown -> Start [order 1] : [(Switch == 0||Switch==1||Switch==2)&&(PassengerSwitch==0||PassengerSwitch==1||PassengerSwitch==2)]
  WindowUp -> Start [order 3] : [Switche==0]
  WindowUp -> EmergencyStop [order 1] : [MotorDraw>3]
  Start -> WindowDown [order 6] : [PassengerSwitch==-1 && Position>MinPos && DisableSwitch==0]
  Start -> ExpressDown [order 8] : [PassengerSwitch==-2 && Position>MinPos && DisableSwitch==0]
  ExpressDown -> Start : [ReturnToInitial==-1]
  EmergencyStop -> Start : [ReturnToInitial == -1]{ReturnToInitial=0;}
  Start -> ExpressDown [order 4] : [Switch==-2 && Position>=MinPos]
  data: Switch input; PassengerSwitch input; DisableSwitch input; MaxPos local =5; MinPos local =0; MotorDraw input; Position output =0; ReturnToInitial local =0; Switche local =1

== stateflow chart MBD_Arnav2020b/BMC/AutomatedBMC/Arnav's Subsytem (Interior Lighting and power windows) / InteriorLighting/DoorLightOperations ==
  state On
  state DomeLightInitialization
    entry:
    DomeLightOutput=1;
  state ReadingLightIntialisation
    entry:
    FrontReadingOutput=1;
    RearReadingOutput=1;
  state Off
    entry:
    FrontReadingOutput=0;
    RearReadingOutput=0;
    DomeLightOutput=0;
  (default) -> On
  Off -> On : [DoorStatus==1]
  On -> ReadingLightIntialisation : [DoorStatus==1]
  ReadingLightIntialisation -> DomeLightInitialization [order 2] : [DomeLight_Enable==1]
  DomeLightInitialization -> ReadingLightIntialisation [order 2] : [DomeLight_Enable==0]{DomeLightOutput=0;}
  DomeLightInitialization -> (junction 27) [order 1] : [DoorStatus==0]
  ReadingLightIntialisation -> (junction 27) [order 1] : [DoorStatus==0]
  (junction 27) -> Off : after(3,sec)
  data: FrontReadingOutput output; RearReadingOutput output; DomeLightOutput output; DomeLight_Enable input; DoorStatus input

== stateflow chart MBD_Arnav2020b/BMC/AutomatedBMC/Arnav's Subsytem (Interior Lighting and power windows) / InteriorLighting/InstrumentPanelLight ==
  state On
  state InstrumentClusterInitialization
    during:
    while(Light<IlluminationValue)
    Light = Light+1;
    end
  state Off
    entry:
    Light=0;
  (default) -> On
  Off -> On : [PilotSwitch==1]
  On -> InstrumentClusterInitialization : [PilotSwitch==1]
  InstrumentClusterInitialization -> Off : [PilotSwitch==0]
  data: PilotSwitch input; IlluminationValue input; Light output =0

== stateflow chart MBD_Arnav2020b/BMC/AutomatedBMC/Arnav's Subsytem (Interior Lighting and power windows) /PowerWindow/Chart ==
  state ExpressUp
    during:
    if Position<MaxPos && (Switch ~= -1 || Switch ~=-2)
    Position=Position+1;
    else
    ReturnToInitial=1;
    end
    exit:
    ReturnToInitial=0;
  state WindowUp
    during:
    if Position<MaxPos
    Position=Position+1;
    else
    Switche=0;
    end
    exit:
    Switche=1;
  state Start
  state EmergencyStop
    during:
    if Position>MinPos
    Position=Position-1;
    else
    ReturnToInitial =-1;
    end
  state WindowDown
    during:
    if Position>MinPos
    Position=Position-1;
    else
    Switche=0;
    end
    exit:
    Switche=-1;
  state ExpressDown
    entry:
    if MotorDraw>3
    while(Position>MinPos)
    Position=Position-1;
    end
    end
    during:
    if Position>MinPos && (Switch~= 1 || Switch ~=2)
    Position=Position-1;
    else
    ReturnToInitial =-1;
    end
    exit:
    ReturnToInitial=0;
  Start -> EmergencyStop [order 5] : [MotorDraw>3]
  ExpressUp -> Start [order 2] : [ReturnToInitial==1]
  Start -> ExpressUp [order 4] : [Switch==2]
  WindowUp -> Start [order 3] : [Switche==0]
  (default) -> Start
  Start -> WindowUp [order 1] : [Switch == 1&& Position<MaxPos]
  ExpressUp -> EmergencyStop [order 1] : [MotorDraw>3]
  WindowUp -> Start [order 2] : [Switch==0]
  ExpressDown -> Start : [ReturnToInitial==-1]
  Start -> ExpressDown [order 3] : [Switch==-2]
  WindowDown -> Start [order 2] : [Switche==0]
  EmergencyStop -> Start : [ReturnToInitial==-1]{ReturnToInitial==0}
  WindowDown -> Start [order 1] : [Switch==0]
  Start -> WindowDown [order 2] : [Switch==-1&& Position>MinPos ]
  WindowUp -> EmergencyStop [order 1] : [MotorDraw>3]
  data: Switch input; MaxPos local =5; MinPos local =0; MotorDraw input; Position output =0; ReturnToInitial local =0; Switche local =1

== stateflow chart MBD_Arnav2020b/BMC/AutomatedBMC/Arnav's Subsytem (Interior Lighting and power windows) /PowerWindow/Chart1 ==
  state ExpressUp
    during:
    if Position<MaxPos && (Switch ~= -1 || Switch ~=-2 || PassengerSwitch ~=-1 || PassengerSwitch~=-2)
    Position=Position+1;
    else
    ReturnToInitial=1;
    end
    exit:
    ReturnToInitial=0;
  state WindowDown
    during:
    if Position>MinPos
    Position=Position-1;
    else
    Switche=0;
    end
    exit:
    Switche=-1;
  state Start
  state WindowUp
    during:
    if Position<MaxPos
    Position=Position+1;
    else
    Switche=0;
    end
    exit:
    Switche=1;
  state EmergencyStop
    during:
    if Position>MinPos
    Position=Position-1;
    else
    ReturnToInitial =-1;
    end
  state ExpressDown
    during:
    if Position>MinPos && (Switch~= 1 || Switch ~=2 || PassengerSwitch ~=1 || PassengerSwitch~=2)
    Position=Position-1;
    else
    ReturnToInitial =-1;
    end
    exit:
    ReturnToInitial=0;
  ExpressUp -> EmergencyStop [order 1] : [MotorDraw>3]
  Start -> ExpressUp [order 7] : [PassengerSwitch==2 && Position<MaxPos && DisableSwitch==0]
  ExpressUp -> Start [order 2] : [ReturnToInitial==1]
  Start -> ExpressUp [order 3] : [Switch==2&& Position<=MaxPos]
  Start -> EmergencyStop [order 9] : [MotorDraw>3]
  (default) -> Start
  Start -> WindowUp [order 5] : [PassengerSwitch==1 && Position<MaxPos && DisableSwitch==0]
  WindowDown -> Start [order 2] : [Switche==0]
  Start -> WindowUp [order 1] : [Switch == 1&& Position<=MaxPos]
  WindowUp -> Start [order 2] : [(Switch == 0||Switch == -1 || Switch ==-2)&&(PassengerSwitch==0||PassengerSwitch==-1||PassengerSwitch==-2)]
  Start -> WindowDown [order 2] : [Switch==-1&& Position>=MinPos ]
  WindowDown -> Start [order 1] : [(Switch == 0||Switch==1||Switch==2)&&(PassengerSwitch==0||PassengerSwitch==1||PassengerSwitch==2)]
  WindowUp -> Start [order 3] : [Switche==0]
  WindowUp -> EmergencyStop [order 1] : [MotorDraw>3]
  Start -> WindowDown [order 6] : [PassengerSwitch==-1 && Position>MinPos && DisableSwitch==0]
  Start -> ExpressDown [order 8] : [PassengerSwitch==-2 && Position>MinPos && DisableSwitch==0]
  ExpressDown -> Start : [ReturnToInitial==-1]
  EmergencyStop -> Start : [ReturnToInitial == -1]{ReturnToInitial=0;}
  Start -> ExpressDown [order 4] : [Switch==-2 && Position>=MinPos]
  data: Switch input; PassengerSwitch input; DisableSwitch input; MaxPos local =5; MinPos local =0; MotorDraw input; Position output =0; ReturnToInitial local =0; Switche local =1

== stateflow chart MBD_Arnav2020b/BMC/AutomatedBMC/Arnav's Subsytem (Interior Lighting and power windows) /PowerWindow/Chart2 ==
  state ExpressUp
    during:
    if Position<MaxPos && (Switch ~= -1 || Switch ~=-2 || PassengerSwitch ~=-1 || PassengerSwitch~=-2)
    Position=Position+1;
    else
    ReturnToInitial=1;
    end
    exit:
    ReturnToInitial=0;
  state WindowDown
    during:
    if Position>MinPos
    Position=Position-1;
    else
    Switche=0;
    end
    exit:
    Switche=-1;
  state Start
  state WindowUp
    during:
    if Position<MaxPos
    Position=Position+1;
    else
    Switche=0;
    end
    exit:
    Switche=1;
  state EmergencyStop
    during:
    if Position>MinPos
    Position=Position-1;
    else
    ReturnToInitial =-1;
    end
  state ExpressDown
    during:
    if Position>MinPos && (Switch~= 1 || Switch ~=2 || PassengerSwitch ~=1 || PassengerSwitch~=2)
    Position=Position-1;
    else
    ReturnToInitial =-1;
    end
    exit:
    ReturnToInitial=0;
  ExpressUp -> EmergencyStop [order 1] : [MotorDraw>3]
  Start -> ExpressUp [order 7] : [PassengerSwitch==2 && Position<MaxPos && DisableSwitch==0]
  ExpressUp -> Start [order 2] : [ReturnToInitial==1]
  Start -> ExpressUp [order 3] : [Switch==2&& Position<=MaxPos]
  Start -> EmergencyStop [order 9] : [MotorDraw>3]
  (default) -> Start
  Start -> WindowUp [order 5] : [PassengerSwitch==1 && Position<MaxPos && DisableSwitch==0]
  WindowDown -> Start [order 2] : [Switche==0]
  Start -> WindowUp [order 1] : [Switch == 1&& Position<=MaxPos]
  WindowUp -> Start [order 2] : [(Switch == 0||Switch == -1 || Switch ==-2)&&(PassengerSwitch==0||PassengerSwitch==-1||PassengerSwitch==-2)]
  Start -> WindowDown [order 2] : [Switch==-1&& Position>=MinPos ]
  WindowDown -> Start [order 1] : [(Switch == 0||Switch==1||Switch==2)&&(PassengerSwitch==0||PassengerSwitch==1||PassengerSwitch==2)]
  WindowUp -> Start [order 3] : [Switche==0]
  WindowUp -> EmergencyStop [order 1] : [MotorDraw>3]
  Start -> WindowDown [order 6] : [PassengerSwitch==-1 && Position>MinPos && DisableSwitch==0]
  Start -> ExpressDown [order 8] : [PassengerSwitch==-2 && Position>MinPos && DisableSwitch==0]
  ExpressDown -> Start : [ReturnToInitial==-1]
  EmergencyStop -> Start : [ReturnToInitial == -1]{ReturnToInitial=0;}
  Start -> ExpressDown [order 4] : [Switch==-2 && Position>=MinPos]
  data: Switch input; PassengerSwitch input; DisableSwitch input; MaxPos local =5; MinPos local =0; MotorDraw input; Position output =0; ReturnToInitial local =0; Switche local =1

== stateflow chart MBD_Arnav2020b/BMC/AutomatedBMC/Arnav's Subsytem (Interior Lighting and power windows) /PowerWindow/Chart3 ==
  state ExpressUp
    during:
    if Position<MaxPos && (Switch ~= -1 || Switch ~=-2 || PassengerSwitch ~=-1 || PassengerSwitch~=-2)
    Position=Position+1;
    else
    ReturnToInitial=1;
    end
    exit:
    ReturnToInitial=0;
  state WindowDown
    during:
    if Position>MinPos
    Position=Position-1;
    else
    Switche=0;
    end
    exit:
    Switche=-1;
  state Start
  state WindowUp
    during:
    if Position<MaxPos
    Position=Position+1;
    else
    Switche=0;
    end
    exit:
    Switche=1;
  state EmergencyStop
    during:
    if Position>MinPos
    Position=Position-1;
    else
    ReturnToInitial =-1;
    end
  state ExpressDown
    during:
    if Position>MinPos && (Switch~= 1 || Switch ~=2 || PassengerSwitch ~=1 || PassengerSwitch~=2)
    Position=Position-1;
    else
    ReturnToInitial =-1;
    end
    exit:
    ReturnToInitial=0;
  ExpressUp -> EmergencyStop [order 1] : [MotorDraw>3]
  Start -> ExpressUp [order 7] : [PassengerSwitch==2 && Position<MaxPos && DisableSwitch==0]
  ExpressUp -> Start [order 2] : [ReturnToInitial==1]
  Start -> ExpressUp [order 3] : [Switch==2&& Position<=MaxPos]
  Start -> EmergencyStop [order 9] : [MotorDraw>3]
  (default) -> Start
  Start -> WindowUp [order 5] : [PassengerSwitch==1 && Position<MaxPos && DisableSwitch==0]
  WindowDown -> Start [order 2] : [Switche==0]
  Start -> WindowUp [order 1] : [Switch == 1&& Position<=MaxPos]
  WindowUp -> Start [order 2] : [(Switch == 0||Switch == -1 || Switch ==-2)&&(PassengerSwitch==0||PassengerSwitch==-1||PassengerSwitch==-2)]
  Start -> WindowDown [order 2] : [Switch==-1&& Position>=MinPos ]
  WindowDown -> Start [order 1] : [(Switch == 0||Switch==1||Switch==2)&&(PassengerSwitch==0||PassengerSwitch==1||PassengerSwitch==2)]
  WindowUp -> Start [order 3] : [Switche==0]
  WindowUp -> EmergencyStop [order 1] : [MotorDraw>3]
  Start -> WindowDown [order 6] : [PassengerSwitch==-1 && Position>MinPos && DisableSwitch==0]
  Start -> ExpressDown [order 8] : [PassengerSwitch==-2 && Position>MinPos && DisableSwitch==0]
  ExpressDown -> Start : [ReturnToInitial==-1]
  EmergencyStop -> Start : [ReturnToInitial == -1]{ReturnToInitial=0;}
  Start -> ExpressDown [order 4] : [Switch==-2 && Position>=MinPos]
  data: Switch input; PassengerSwitch input; DisableSwitch input; MaxPos local =5; MinPos local =0; MotorDraw input; Position output =0; ReturnToInitial local =0; Switche local =1

== stateflow chart MBD_Arnav2020b/BMC/ManualTesting/Manual Testing Arnav/BMC/ManualInteriorLighting/DoorLightOperations ==
  state On
  state DomeLightInitialization
    entry:
    DomeLightOutput=1;
  state ReadingLightIntialisation
    entry:
    FrontReadingOutput=1;
    RearReadingOutput=1;
  state Off
    entry:
    FrontReadingOutput=0;
    RearReadingOutput=0;
    DomeLightOutput=0;
  (default) -> On
  Off -> On : [DoorStatus==1]
  On -> ReadingLightIntialisation : [DoorStatus==1]
  ReadingLightIntialisation -> DomeLightInitialization [order 2] : [DomeLight_Enable==1]
  DomeLightInitialization -> ReadingLightIntialisation [order 2] : [DomeLight_Enable==0]{DomeLightOutput=0;}
  DomeLightInitialization -> (junction 27) [order 1] : [DoorStatus==0]
  ReadingLightIntialisation -> (junction 27) [order 1] : [DoorStatus==0]
  (junction 27) -> Off : after(3,sec)
  data: FrontReadingOutput output; RearReadingOutput output; DomeLightOutput output; DomeLight_Enable input; DoorStatus input

== stateflow chart MBD_Arnav2020b/BMC/ManualTesting/Manual Testing Arnav/BMC/ManualInteriorLighting/InstrumentPanelLight ==
  state On
  state InstrumentClusterInitialization
    during:
    while(Light<IlluminationValue)
    Light = Light+1;
    end
  state Off
    entry:
    Light=0;
  (default) -> On
  Off -> On : [PilotSwitch==1]
  On -> InstrumentClusterInitialization : [PilotSwitch==1]
  InstrumentClusterInitialization -> Off : [PilotSwitch==0]
  data: PilotSwitch input; IlluminationValue input; Light output =0

== stateflow chart MBD_Arnav2020b/BMC/ManualTesting/Manual Testing Arnav/BMC/ManualInteriorLighting/TrueFalse ==
  state TrueFalse
    during:
    if inp==true
    out=1;
    elseif inp == false
    out=0;
    end
  (default) -> TrueFalse
  data: out output; inp input

== stateflow chart MBD_Arnav2020b/BMC/ManualTesting/Manual Testing Arnav/BMC/ManualInteriorLighting/TrueFalse1 ==
  state TrueFalse
    during:
    if inp==true
    out=1;
    elseif inp == false
    out=0;
    end
  (default) -> TrueFalse
  data: out output; inp input
